simulink model "Induction_motor_drive"  (R2025a)
settings: Solver=ode45  StartTime=0.0  StopTime=1  RelTol=1e-3  EnableMultiTasking=on
libraries: spsIGBTDiodeLib x6, dspfdesign x3, spsCurrentMeasurementLib x3, spsVoltageMeasurementLib x3, spsGroundLib x1, simulink x1, spsDCVoltageSourceLib x1, sps_lib x1
settings Model: Creator=Cheku  LastModifiedBy=vijay
settings SolverCC: AlgebraicLoopSolver=TrustRegion
settings DataIOCC: LimitDataPoints=on  SaveFormat=Array  SignalLoggingSaveFormat=ModelDataLogs  ReturnWorkspaceOutputs=off
settings OptimizationCC: ExpressionDepthLimit=2147483647.0  InitFltsAndDblsToZero=on  LifeSpan=inf
settings DebuggingCC: UnderspecifiedInitializationDetection=Classic  MergeDetectMultiDrivingBlocksExec=none  SolverPrmCheckMsg=warning  FcnCallInpInsideContextMsg=warning  UnconnectedInputMsg=warning  UnconnectedOutputMsg=warning  UnconnectedLineMsg=warning  StateNameClashWarn=warning  SFUnexpectedBacktrackingDiag=warning  SFNoUnconditionalDefaultTransitionDiag=warning  SFExecutionAtInitializationDiag=none  ArithmeticOperatorsInVariantConditions=warning
settings HardwareCC: ProdBitPerPointer=32.0  ProdBitPerSizeT=32.0  ProdBitPerPtrDiffT=32.0  ProdLargestAtomicFloat=None  ProdIntDivRoundTo=Undefined  ProdEndianess=Unspecified  ProdWordSize=32.0  ProdHWDeviceType=32-bit Generic
settings ModelReferenceCC: PropagateSignalLabelsOutOfModel=off
settings SFSimCC: SimUseLocalCustomCode=off  CustomCodeUndefinedFunction=UseInterfaceOnly
settings RTWCC: RTWUseLocalCustomCode=off  GPUComputeCapability=3.5
settings CodeAppCC: StateflowObjectComments=on
settings GRTTargetCC: TargetLangStandard=C89/C90 (ANSI)  CombineOutputUpdateFcns=off  GRTInterface=on
settings ConfigComp: CovMetricSettings=dw  CovSaveCumulativeToWorkspaceVar=on  CovSaveSingleToWorkspaceVar=on  CovExternalEMLEnable=off

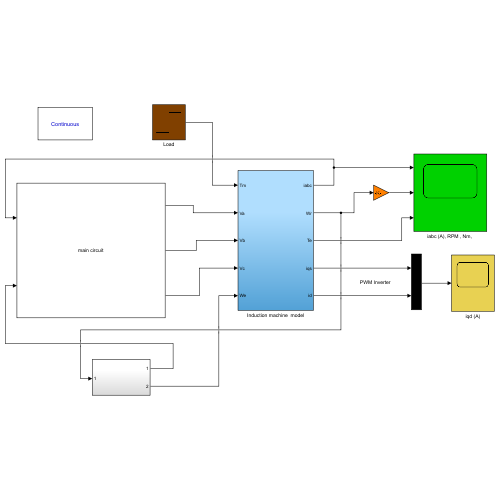
[thumbnail: Simulink's stored preview of the top-level diagram]
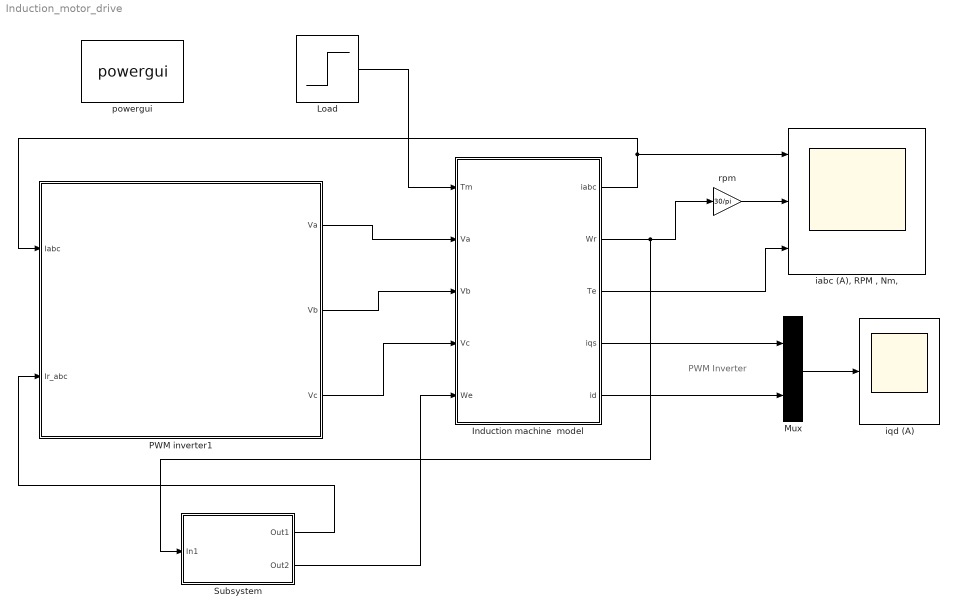
== system Induction_motor_drive ==
  note: PWM Inverter
  " rpm" : Gain  Gain=30/pi
  Induction machine  model : Subsystem
  Load : Step  Time=0  Before=0.025  After=5.00  SampleTime=0
  Mux : Mux  Inputs=2
  PWM inverter1 : Subsystem
      mask Display: disp('main circuit')
  Subsystem : Subsystem
  "iabc (A), RPM , Nm, " : Scope  NumInputPorts=3
      settings: TimeSpan=0.1  ActiveDisplayYMinimum=-681.97623  ActiveDisplayYMaximum=702.05177  DataLoggingVariableName=ScopeData9
  iqd (A) : Scope
      settings: ActiveDisplayYMinimum=-491.36775454277125  ActiveDisplayYMaximum=643.61004745722926  DataLoggingVariableName=ScopeData3
  powergui : sps_lib/powergui  SimulationMode=Continuous  SampleTime=50e-6  frequency=60  Iterations=50  frequencyindice=0  Pbase=100e6  ErrMax=1e-4  UnitsV=kV  UnitsW=MW  buscounter=0  FunctionMessages=off  echomessages=off  EnableUseOfTLC=off  CurrentSourceSwitches=on  DisableSnubberDevices=off  DisableRonSwitches=off  DisableVfSwitches=off  DisplayEquations=off  AutomaticDiscreteSolvers=off  SolverType=Tustin/Backward Euler (TBE)  Interpol=off  ExternalGateDelay=off  methode=off  Ts=0  x0status=blocks  SPID=off  SwTol=0  HookPort=off  NonlinearTolerance=1e-4  nMaxIteration=100  ContinueOnMaxIteration=off  RestoreLinks=warning  ResistiveCurrentMeasurement=off  Frange=[0:2:500]  Ylog=off  Xlog=on  ShowGrid=off  save=off  variable=ZData  structure=0  ZoomFFT=on  StartTime=0.0  cycles=1  DisplayStyle=1  fundamental=60  FreqAxis=off  MaxFrequency=1000  frequencyindicesteady=1  RmsSteady=1  display=off
  wires:
  PWM inverter1/1(Va) -> Induction machine  model/2(Va)
  Load/1 -> Induction machine  model/1(Tm)
  PWM inverter1/2(Vb) -> Induction machine  model/3(Vb)
  PWM inverter1/3(Vc) -> Induction machine  model/4(Vc)
  Subsystem/1(Out1) -> PWM inverter1/2(Ir_abc)
  Induction machine  model/1(iabc) -> "iabc (A), RPM , Nm, "/1, PWM inverter1/1(Iabc)
  Induction machine  model/2(Wr) -> Subsystem/1(In1), " rpm"/1
  Mux/1 -> iqd (A)/1
  Induction machine  model/4(iqs) -> Mux/1
  Induction machine  model/5(id) -> Mux/2
  Induction machine  model/3(Te) -> "iabc (A), RPM , Nm, "/3
  " rpm"/1 -> "iabc (A), RPM , Nm, "/2
  Subsystem/2(Out2) -> Induction machine  model/5(We)

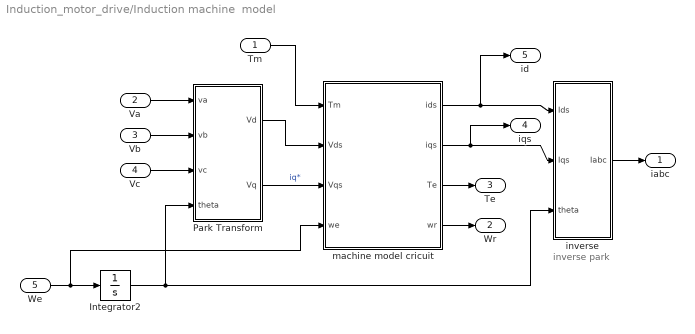
== system Induction_motor_drive/Induction machine  model ==
  note: inverse park
  Tm : Inport
  Va : Inport  Port=2
  Vb : Inport  Port=3
  Vc : Inport  Port=4
  We : Inport  Port=5
  Integrator2 : Integrator
  Park Transform : Subsystem
  "inverse " : Subsystem
  "machine model cricuit " : Subsystem
  iabc : Outport
  Wr : Outport  Port=2
  Te : Outport  Port=3
  iqs : Outport  Port=4
  id : Outport  Port=5
  wires:
  "machine model cricuit "/1(ids) -> "inverse "/1(Ids), id/1
  "machine model cricuit "/2(iqs) -> "inverse "/2(Iqs), iqs/1
  Park Transform/2(Vq) -> "machine model cricuit "/3(Vqs)  "iq*"
  Park Transform/1(Vd) -> "machine model cricuit "/2(Vds)
  Va/1 -> Park Transform/1(va)
  Vb/1 -> Park Transform/2(vb)
  Vc/1 -> Park Transform/3(vc)
  Tm/1 -> "machine model cricuit "/1(Tm)
  "inverse "/1(Iabc) -> iabc/1
  "machine model cricuit "/3(Te) -> Te/1
  We/1 -> Integrator2/1, "machine model cricuit "/4(we)
  "machine model cricuit "/4(wr) -> Wr/1
  Integrator2/1 -> "inverse "/3(theta), Park Transform/4(theta)

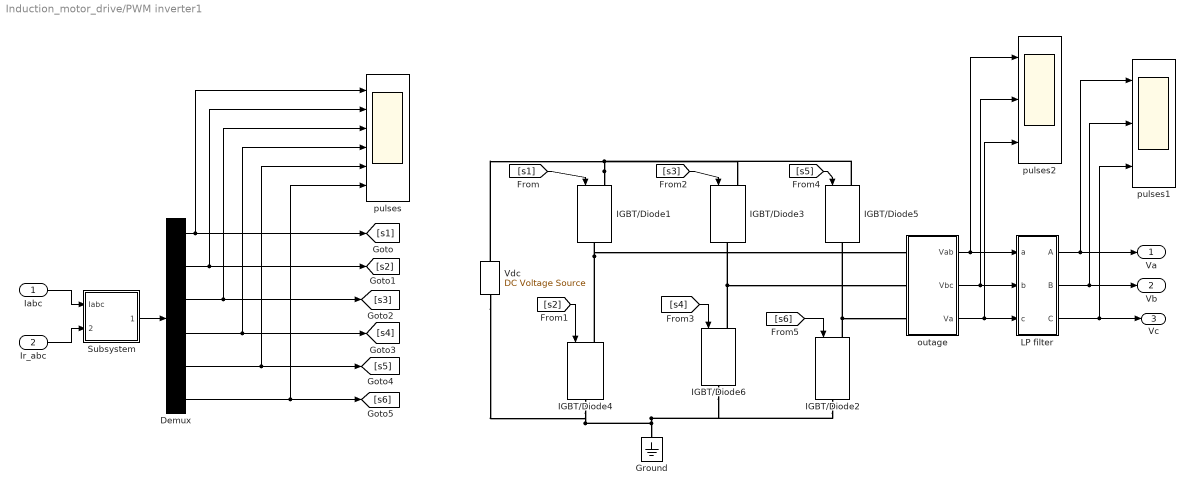
== system Induction_motor_drive/PWM inverter1 ==
  Iabc : Inport
  Ir_abc : Inport  Port=2
  Demux : Demux  Outputs=6
  Ground : spsGroundLib/Ground  LConnTagsString=a
  IGBT/Diode{1..6} (6 alike) : spsIGBTDiodeLib/IGBT//Diode  Ron=1e-3  Rs=1e5  Cs=inf  Measurements=off
  LP filter : Subsystem
  Subsystem : Subsystem
  Vdc : spsDCVoltageSourceLib/DC Voltage Source  Amplitude=283  Measurements=None
  outage : Subsystem
  pulses : Scope  NumInputPorts=6
      settings: ActiveDisplayYMinimum=-0.12499999999999997  ActiveDisplayYMaximum=1.125
  pulses1 : Scope  NumInputPorts=3
      settings: ActiveDisplayYMinimum=-143.13602  ActiveDisplayYMaximum=143.36169  DataLoggingVariableName=ScopeData2
  pulses2 : Scope  NumInputPorts=3
      settings: ActiveDisplayYMinimum=-353.74999292483255  ActiveDisplayYMaximum=353.74999292541224  DataLoggingVariableName=ScopeData4
  Va : Outport
  Vb : Outport  Port=2
  Vc : Outport  Port=3
  wires:
  Iabc/1 -> Subsystem/1(Iabc)
  Ir_abc/1 -> Subsystem/2(Ir_abc)
  Subsystem/1(pulses) -> Demux/1
  Demux/1 -> [s1], pulses/1
  [s1] -> IGBT/Diode1/1
  Demux/2 -> [s2], pulses/2
  [s2] -> IGBT/Diode4/1
  [s3] -> IGBT/Diode3/1
  Demux/3 -> [s3], pulses/3
  [s4] -> IGBT/Diode6/1
  Demux/4 -> [s4], pulses/4
  [s5] -> IGBT/Diode5/1
  [s6] -> IGBT/Diode2/1
  Demux/5 -> [s5], pulses/5
  Demux/6 -> [s6], pulses/6
  outage/1(Vab) -> LP filter/1(a), pulses2/1
  outage/2(Vbc) -> LP filter/2(b), pulses2/2
  outage/3(Va) -> LP filter/3(c), pulses2/3
  LP filter/1(A) -> Va/1, pulses1/1
  LP filter/2(B) -> Vb/1, pulses1/2
  LP filter/3(C) -> Vc/1, pulses1/3
  connections:
  IGBT/Diode1/LConn1 -- Vdc/RConn1 -- IGBT/Diode3/LConn1 -- IGBT/Diode5/LConn1
  IGBT/Diode4/LConn1 -- IGBT/Diode1/RConn1 -- outage/LConn1
  IGBT/Diode2/LConn1 -- IGBT/Diode5/RConn1 -- outage/LConn3
  Ground/LConn1 -- IGBT/Diode2/RConn1 -- IGBT/Diode6/RConn1 -- Vdc/LConn1 -- IGBT/Diode4/RConn1
  IGBT/Diode6/LConn1 -- outage/LConn2 -- IGBT/Diode3/RConn1

== system Induction_motor_drive/Subsystem ==
  In1 : Inport
  Integrator2 : Integrator
  Ref. Speed (rpm) : Constant  Value=1500
  "Ref. iabc " : Subsystem
  Sum : Sum  Inputs=+-  InputSameDT=on  SaturateOnIntegerOverflow=on  OutDataTypeStr=Inherit: Same as first input
  Sum2 : Sum
  Vector  control : Subsystem
  flux controller : Subsystem
  iqref1 : Subsystem  mask(PI Controller){I=2.5, P=5, sat=[ -30 30]}
      mask prompts: I "Integral"; P "Proportional:"; sat "Minimum and maximum outputs:"
      mask init:
      | min=sat(1);max=sat(2);
      mask Display: disp('PI')
  rad/sec : Gain  Gain=pi/30
  Out1 : Outport
  Out2 : Outport  Port=2
  wires:
  Ref. Speed (rpm)/1 -> rad/sec/1
  Sum/1 -> iqref1/1(In_1)
  rad/sec/1 -> Sum/1
  Vector  control/1(is*) -> "Ref. iabc "/1(is*)
  iqref1/1(Out_1) -> Vector  control/1(Te*)
  flux controller/1(Yr*) -> Vector  control/2(Yr)
  Sum2/1 -> Integrator2/1, Out2/1
  Integrator2/1 -> "Ref. iabc "/2(theta)
  Vector  control/2(wsl) -> Sum2/1
  In1/1 -> Sum2/2, Sum/2, flux controller/1(Wr)
  "Ref. iabc "/1(irabc) -> Out1/1

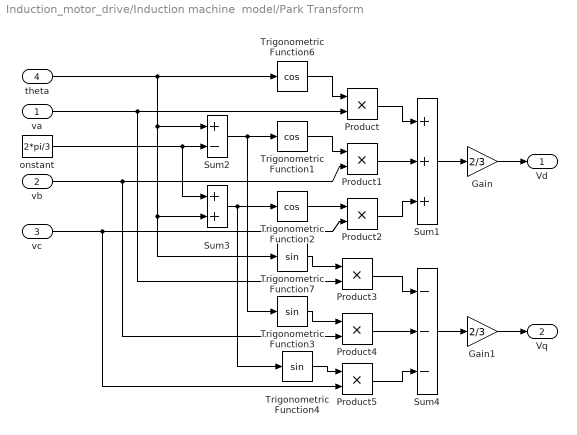
== system Induction_motor_drive/Induction machine  model/Park Transform ==
  va : Inport
  vb : Inport  Port=2
  vc : Inport  Port=3
  theta : Inport  Port=4
  Gain : Gain  Gain=2/3
  Gain1 : Gain  Gain=2/3
  Product{,1..5} (6 alike) : Product  RndMeth=Zero
  Sum1 : Sum  Inputs=+++  InputSameDT=on  SaturateOnIntegerOverflow=on  OutDataTypeStr=Inherit: Same as first input
  Sum2 : Sum  Inputs=+-  InputSameDT=on  SaturateOnIntegerOverflow=on  OutDataTypeStr=Inherit: Same as first input
  Sum3 : Sum  InputSameDT=on  SaturateOnIntegerOverflow=on  OutDataTypeStr=Inherit: Same as first input
  Sum4 : Sum  Inputs=---  InputSameDT=on  SaturateOnIntegerOverflow=on  OutDataTypeStr=Inherit: Same as first input
  Trigonometric Function1 : Trigonometry  Operator=cos
  Trigonometric Function2 : Trigonometry  Operator=cos
  Trigonometric Function3 : Trigonometry
  Trigonometric Function4 : Trigonometry
  Trigonometric Function6 : Trigonometry  Operator=cos
  Trigonometric Function7 : Trigonometry
  onstant : Constant  Value=2*pi/3
  Vd : Outport
  Vq : Outport  Port=2
  wires:
  Gain1/1 -> Vq/1
  Sum4/1 -> Gain1/1
  Product5/1 -> Sum4/3
  Trigonometric Function4/1 -> Product5/1
  Product4/1 -> Sum4/2
  Trigonometric Function3/1 -> Product4/1
  Product3/1 -> Sum4/1
  Trigonometric Function7/1 -> Product3/1
  Gain/1 -> Vd/1
  Sum1/1 -> Gain/1
  Product2/1 -> Sum1/3
  vc/1 -> Product5/2, Product2/2
  Trigonometric Function2/1 -> Product2/1
  Sum3/1 -> Trigonometric Function4/1, Trigonometric Function2/1
  Product1/1 -> Sum1/2
  vb/1 -> Product4/2, Product1/2
  Trigonometric Function1/1 -> Product1/1
  Sum2/1 -> Trigonometric Function3/1, Trigonometric Function1/1
  onstant/1 -> Sum3/1, Sum2/2
  Product/1 -> Sum1/1
  va/1 -> Product3/2, Product/2
  Trigonometric Function6/1 -> Product/1
  theta/1 -> Sum3/2, Trigonometric Function7/1, Sum2/1, Trigonometric Function6/1

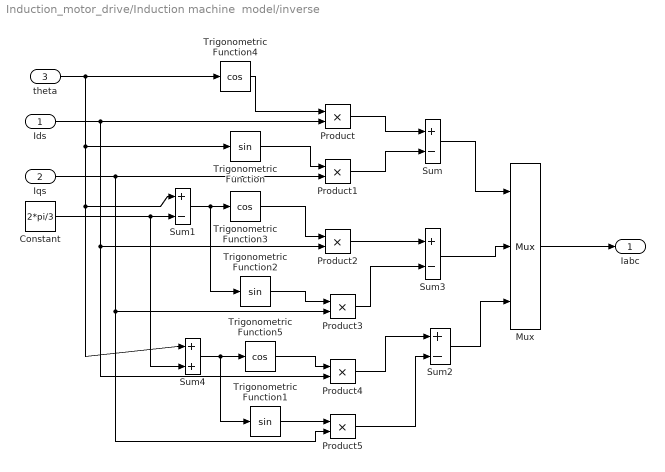
== system Induction_motor_drive/Induction machine  model/inverse  ==
  Ids : Inport
  Iqs : Inport  Port=2
  theta : Inport  Port=3
  Constant : Constant  Value=2*pi/3
  Mux : Mux  Inputs=3
  Product{,1..5} (6 alike) : Product  RndMeth=Zero
  Sum{,1..3} (4 alike) : Sum  Inputs=+-
  Sum4 : Sum  Inputs=|++
  Trigonometric Function : Trigonometry
  Trigonometric Function1 : Trigonometry
  Trigonometric Function2 : Trigonometry
  Trigonometric Function3 : Trigonometry  Operator=cos
  Trigonometric Function4 : Trigonometry  Operator=cos
  Trigonometric Function5 : Trigonometry  Operator=cos
  Iabc : Outport
  wires:
  Mux/1 -> Iabc/1
  Sum/1 -> Mux/1
  Sum3/1 -> Mux/2
  Sum2/1 -> Mux/3
  Product5/1 -> Sum2/2
  Product4/1 -> Sum2/1
  Trigonometric Function1/1 -> Product5/1
  Trigonometric Function5/1 -> Product4/1
  Sum4/1 -> Trigonometric Function1/1, Trigonometric Function5/1
  Product3/1 -> Sum3/2
  Trigonometric Function2/1 -> Product3/1
  Product2/1 -> Sum3/1
  Trigonometric Function3/1 -> Product2/1
  Sum1/1 -> Trigonometric Function2/1, Trigonometric Function3/1
  Constant/1 -> Sum4/2, Sum1/2
  Product1/1 -> Sum/2
  Product/1 -> Sum/1
  Iqs/1 -> Product5/2, Product3/2, Product1/2
  Trigonometric Function/1 -> Product1/1
  Ids/1 -> Product4/2, Product2/2, Product/2
  theta/1 -> Trigonometric Function/1, Sum4/1, Sum1/1, Trigonometric Function4/1
  Trigonometric Function4/1 -> Product/1

== system Induction_motor_drive/Induction machine  model/machine model cricuit  ==
  Tm : Inport
  Vds : Inport  Port=2
  Vqs : Inport  Port=3
  we : Inport  Port=4
  Saturation : Saturate  UpperLimit=5  LowerLimit=0
  Subsyste1 : Subsystem
  Subsystem : Subsystem
  Subsystem1 : Subsystem
  ids crt : Subsystem
  iqs crt : Subsystem
  ids : Outport
  iqs : Outport  Port=2
  Te : Outport  Port=3
  wr : Outport  Port=4
  wires:
  ids crt/1(ids) -> Subsystem/2(ids), Subsyste1/1(ids), iqs crt/4(ids), ids/1
  iqs crt/1(iqs) -> Subsystem/5(iqs), Subsystem1/4(iqs), ids crt/4(iqs), iqs/1
  Subsystem/2(wr) -> wr/1, iqs crt/6(Wr), ids crt/6(Wr), Subsyste1/3(Wr), Subsystem1/3(Wr)
  Subsystem1/1(Yqr) -> Subsystem/3(yqr), ids crt/2(Yqr), Subsyste1/4(Yqr), iqs crt/3(Yqr)
  Subsyste1/1(Ydr) -> ids crt/3(Ydr), Subsystem1/1(Ydr), Subsystem/4(ydr), iqs crt/2(Ydr)
  Tm/1 -> Subsystem/1(TM)
  we/1 -> Subsyste1/2(We), ids crt/5(We), Subsystem1/2(We), iqs crt/5(We)
  Vqs/1 -> iqs crt/1(Vqs)
  Vds/1 -> ids crt/1(Vds)
  Subsystem/1(Te) -> Saturation/1
  Saturation/1 -> Te/1

== system Induction_motor_drive/PWM inverter1/LP filter ==
  a : Inport
  b : Inport  Port=2
  c : Inport  Port=3
  Analog Filter Desg : dspfdesign/Analog Filter Design  method=Butterworth  filttype=Lowpass  N=3  Wlo=12566.3706  Whi=80  Rp=3  Rs=5
  Analog Filter Desg1 : dspfdesign/Analog Filter Design  method=Butterworth  filttype=Lowpass  N=3  Wlo=12566.3706  Whi=80  Rp=3  Rs=5
  Analog Filter Desg2 : dspfdesign/Analog Filter Design  method=Butterworth  filttype=Lowpass  N=3  Wlo=12566.3706  Whi=80  Rp=3  Rs=5
  A : Outport
  B : Outport  Port=2
  C : Outport  Port=3
  wires:
  a/1 -> Analog Filter Desg/1
  Analog Filter Desg/1 -> A/1
  b/1 -> Analog Filter Desg1/1
  Analog Filter Desg1/1 -> B/1
  c/1 -> Analog Filter Desg2/1
  Analog Filter Desg2/1 -> C/1

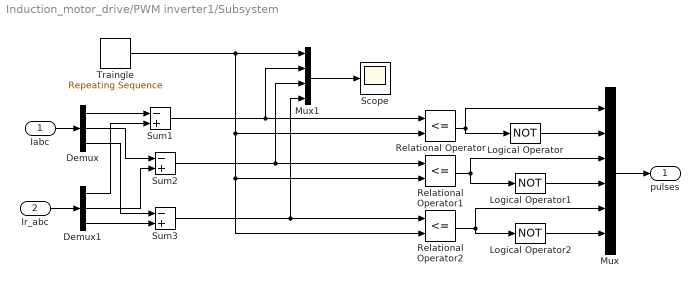
== system Induction_motor_drive/PWM inverter1/Subsystem ==
  Iabc : Inport
  Ir_abc : Inport  Port=2
  Demux : Demux  Outputs=3
  Demux1 : Demux  Outputs=3
  Logical Operator : Logic  Operator=NOT
  Logical Operator1 : Logic  Operator=NOT
  Logical Operator2 : Logic  Operator=NOT
  Mux : Mux  Inputs=6
  Mux1 : Mux
  Relational Operator : RelationalOperator  Operator=<=  OutDataTypeStr=boolean  InputSameDT=off
  Relational Operator1 : RelationalOperator  Operator=<=  OutDataTypeStr=boolean  InputSameDT=off
  Relational Operator2 : RelationalOperator  Operator=<=  OutDataTypeStr=boolean  InputSameDT=off
  Scope : Scope
      settings: ActiveDisplayYMinimum=-124.55267  ActiveDisplayYMaximum=124.74286  DataLoggingVariableName=ScopeData11
  Sum1 : Sum  Inputs=-+  InputSameDT=on  SaturateOnIntegerOverflow=on  OutDataTypeStr=Inherit: Same as first input
  Sum2 : Sum  Inputs=-+  InputSameDT=on  SaturateOnIntegerOverflow=on  OutDataTypeStr=Inherit: Same as first input
  Sum3 : Sum  Inputs=-+  InputSameDT=on  SaturateOnIntegerOverflow=on  OutDataTypeStr=Inherit: Same as first input
  Traingle : simulink/Sources/Repeating Sequence  rep_seq_t=[0 1/2000/4 3/2000/4 1/2000]  rep_seq_y="[0 -100  100  0]"
  pulses : Outport
  wires:
  Iabc/1 -> Demux/1
  Ir_abc/1 -> Demux1/1
  Demux/1 -> Sum1/1
  Demux1/1 -> Sum1/2
  Demux/2 -> Sum2/1
  Demux1/2 -> Sum2/2
  Demux/3 -> Sum3/1
  Demux1/3 -> Sum3/2
  Relational Operator/1 -> Logical Operator/1, Mux/1
  Logical Operator/1 -> Mux/2
  Relational Operator1/1 -> Mux/3, Logical Operator1/1
  Logical Operator1/1 -> Mux/4
  Relational Operator2/1 -> Logical Operator2/1, Mux/5
  Logical Operator2/1 -> Mux/6
  Mux/1 -> pulses/1
  Sum1/1 -> Relational Operator/1, Mux1/2
  Sum2/1 -> Relational Operator1/1, Mux1/3
  Sum3/1 -> Relational Operator2/1, Mux1/4
  Traingle/1 -> Relational Operator2/2, Relational Operator1/2, Relational Operator/2, Mux1/1
  Mux1/1 -> Scope/1

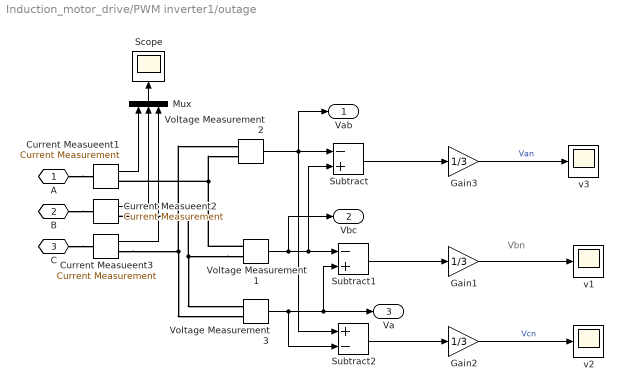
== system Induction_motor_drive/PWM inverter1/outage ==
  note: Vbn
  Current Measueent1 : spsCurrentMeasurementLib/Current Measurement  PhasorSimulation=off  OutputType=Complex  PSBequivalent=0
  Current Measueent2 : spsCurrentMeasurementLib/Current Measurement  PhasorSimulation=off  OutputType=Complex  PSBequivalent=0
  Current Measueent3 : spsCurrentMeasurementLib/Current Measurement  PhasorSimulation=off  OutputType=Complex  PSBequivalent=0
  Gain1 : Gain  Gain=1/3
  Gain2 : Gain  Gain=1/3
  Gain3 : Gain  Gain=1/3
  Mux : Mux  Inputs=3
  Scope : Scope
      settings: ActiveDisplayYMinimum=-3.1169527740766263  ActiveDisplayYMaximum=1.936947616674654
  Subtract : Sum  Inputs=-+
  Subtract1 : Sum  Inputs=-+
  Subtract2 : Sum  Inputs=+-
  Voltage Measurement1 : spsVoltageMeasurementLib/Voltage Measurement  PhasorSimulation=off  OutputType=Complex  PSBequivalent=0
  Voltage Measurement2 : spsVoltageMeasurementLib/Voltage Measurement  PhasorSimulation=off  OutputType=Complex  PSBequivalent=0
  Voltage Measurement3 : spsVoltageMeasurementLib/Voltage Measurement  PhasorSimulation=off  OutputType=Complex  PSBequivalent=0
  v1 : Scope
      settings: ActiveDisplayYMinimum=-283.8728707821619  ActiveDisplayYMaximum=262.14024076146268  DataLoggingVariableName=ScopeData25
  v2 : Scope
      settings: ActiveDisplayYMinimum=-235.8333276306908  ActiveDisplayYMaximum=235.83332850733069  DataLoggingVariableName=ScopeData26
  v3 : Scope
      settings: ActiveDisplayYMinimum=-286.94561491531204  ActiveDisplayYMaximum=259.06749789646426  DataLoggingVariableName=ScopeData27
  A : PMIOPort  Side=Left
  B : PMIOPort  Port=2  Side=Left
  C : PMIOPort  Port=3  Side=Left
  Vab : Outport
  Vbc : Outport  Port=2
  Va : Outport  Port=3
  wires:
  Voltage Measurement2/1 -> Subtract/1, Subtract2/1, Vab/1
  Voltage Measurement1/1 -> Subtract/2, Subtract1/1, Vbc/1
  Current Measueent1/1 -> Mux/1
  Current Measueent2/1 -> Mux/2
  Current Measueent3/1 -> Mux/3
  Mux/1 -> Scope/1
  Subtract/1 -> Gain3/1
  Gain3/1 -> v3/1  "Van"
  Voltage Measurement3/1 -> Subtract2/2, Subtract1/2, Va/1
  Subtract1/1 -> Gain1/1
  Gain1/1 -> v1/1
  Subtract2/1 -> Gain2/1
  Gain2/1 -> v2/1  "Vcn"
  connections:
  Voltage Measurement1/LConn1 -- Current Measueent1/RConn1 -- Voltage Measurement2/LConn2
  Voltage Measurement1/LConn2 -- Current Measueent2/RConn1 -- Voltage Measurement3/LConn1
  Current Measueent3/RConn1 -- Voltage Measurement2/LConn1 -- Voltage Measurement3/LConn2
  A/RConn1 -- Current Measueent1/LConn1
  B/RConn1 -- Current Measueent2/LConn1
  C/RConn1 -- Current Measueent3/LConn1

== system Induction_motor_drive/Subsystem/Ref. iabc  ==
  is* : Inport
  theta : Inport  Port=2
  Constant : Constant  Value=2*pi/3
  Mux1 : Mux  Inputs=3
  Product2 : Product  InputSameDT=on  RndMeth=Zero  SaturateOnIntegerOverflow=on  OutDataTypeStr=Inherit: Same as first input
  Product4 : Product  InputSameDT=on  RndMeth=Zero  SaturateOnIntegerOverflow=on  OutDataTypeStr=Inherit: Same as first input
  Product7 : Product  InputSameDT=on  RndMeth=Zero  SaturateOnIntegerOverflow=on  OutDataTypeStr=Inherit: Same as first input
  Sum2 : Sum  Inputs=+-  InputSameDT=on  SaturateOnIntegerOverflow=on  OutDataTypeStr=Inherit: Same as first input
  Sum4 : Sum  InputSameDT=on  SaturateOnIntegerOverflow=on  OutDataTypeStr=Inherit: Same as first input
  Trigonometric Function1 : Trigonometry  Operator=cos
  Trigonometric Function3 : Trigonometry  Operator=cos
  Trigonometric Function6 : Trigonometry  Operator=cos
  irabc : Outport
  wires:
  theta/1 -> Trigonometric Function6/1, Sum2/1, Sum4/1
  Trigonometric Function6/1 -> Product7/1
  is*/1 -> Product7/2, Product2/2, Product4/2
  Product7/1 -> Mux1/1
  Sum2/1 -> Trigonometric Function1/1
  Trigonometric Function1/1 -> Product2/1
  Product2/1 -> Mux1/2
  Sum4/1 -> Trigonometric Function3/1
  Trigonometric Function3/1 -> Product4/1
  Product4/1 -> Mux1/3
  Mux1/1 -> irabc/1
  Constant/1 -> Sum2/2, Sum4/2

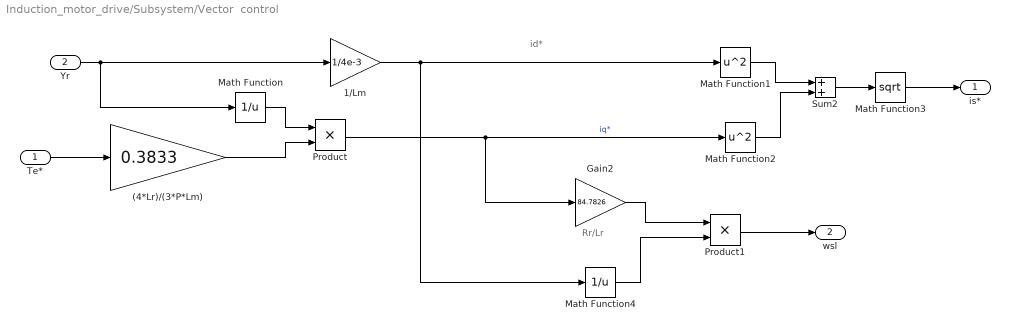
== system Induction_motor_drive/Subsystem/Vector  control ==
  note: id*
  note: Rr/Lr
  Te* : Inport
  Yr : Inport  Port=2
  (4*Lr)/(3*P*Lm) : Gain  Gain=0.3833
  1/Lm : Gain  Gain=1/4e-3
  Gain2 : Gain  Gain=84.7826
  Math Function : Math  Operator=reciprocal  SignedPower=on
  Math Function1 : Math  Operator=square  SignedPower=on
  Math Function2 : Math  Operator=square  SignedPower=on
  Math Function3 : Math  Operator=sqrt  SignedPower=on
  Math Function4 : Math  Operator=reciprocal  SignedPower=on
  Product : Product  RndMeth=Zero
  Product1 : Product  RndMeth=Zero
  Sum2 : Sum
  is* : Outport
  wsl : Outport  Port=2
  wires:
  Yr/1 -> 1/Lm/1, Math Function/1
  Te*/1 -> (4*Lr)/(3*P*Lm)/1
  (4*Lr)/(3*P*Lm)/1 -> Product/2
  Math Function/1 -> Product/1
  Math Function1/1 -> Sum2/1
  Math Function2/1 -> Sum2/2
  Sum2/1 -> Math Function3/1
  Math Function3/1 -> is*/1
  Product/1 -> Gain2/1, Math Function2/1  "iq*"
  1/Lm/1 -> Math Function1/1, Math Function4/1
  Gain2/1 -> Product1/1
  Math Function4/1 -> Product1/2
  Product1/1 -> wsl/1

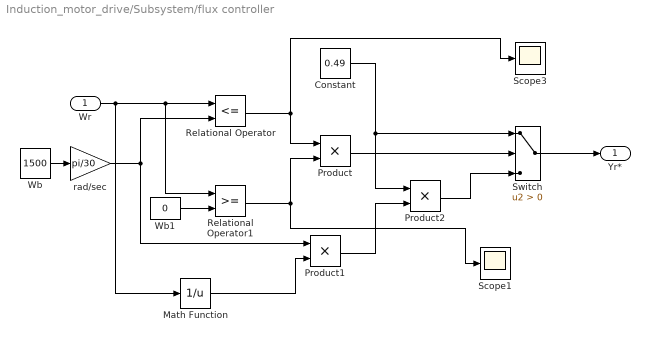
== system Induction_motor_drive/Subsystem/flux controller ==
  Wr : Inport
  Constant : Constant  Value=0.49
  Math Function : Math  Operator=reciprocal  SignedPower=on
  Product : Product  RndMeth=Zero
  Product1 : Product  RndMeth=Zero
  Product2 : Product  RndMeth=Zero
  Relational Operator : RelationalOperator  Operator=<=  OutDataTypeStr=boolean  InputSameDT=off
  Relational Operator1 : RelationalOperator  OutDataTypeStr=boolean  InputSameDT=off
  Scope1 : Scope
      settings: ActiveDisplayYMinimum=-55  ActiveDisplayYMaximum=55  DataLoggingVariableName=ScopeData8
  Scope3 : Scope
      settings: ActiveDisplayYMinimum=-55  ActiveDisplayYMaximum=55  DataLoggingVariableName=ScopeData7
  Switch : Switch  Criteria=u2 > Threshold  SaturateOnIntegerOverflow=off  InputSameDT=off
  Wb : Constant  Value=1500
  Wb1 : Constant  Value=0
  rad/sec : Gain  Gain=pi/30
  Yr* : Outport
  wires:
  Relational Operator/1 -> Product/1, Scope3/1
  Relational Operator1/1 -> Product/2, Scope1/1
  Wr/1 -> Relational Operator/1, Relational Operator1/1, Math Function/1
  Wb/1 -> rad/sec/1
  Product/1 -> Switch/2
  Constant/1 -> Switch/1, Product2/1
  Math Function/1 -> Product1/2
  Product1/1 -> Product2/2
  Product2/1 -> Switch/3
  Switch/1 -> Yr*/1
  Wb1/1 -> Relational Operator1/2
  rad/sec/1 -> Relational Operator/2, Product1/1

== system Induction_motor_drive/Subsystem/iqref1 ==
  In_1 : Inport
  Integral : TransferFcn  Numerator=[I]  Denominator=[1 0]
  Proportional : Gain  Gain=P  SaturateOnIntegerOverflow=on  OutDataTypeStr=Inherit: Same as input  ParamDataTypeStr=Inherit: Same as input
  Saturation : Saturate  UpperLimit=max  LowerLimit=min
  Sum : Sum  InputSameDT=on  SaturateOnIntegerOverflow=on  OutDataTypeStr=Inherit: Same as first input
  Out_1 : Outport  InitialOutput=0
  wires:
  Integral/1 -> Sum/2
  In_1/1 -> Integral/1, Proportional/1
  Proportional/1 -> Sum/1
  Sum/1 -> Saturation/1
  Saturation/1 -> Out_1/1

== system Induction_motor_drive/Induction machine  model/machine model cricuit /Subsyste1 ==
  note: C6 = Lm*Rr/Lr
  note: C5 = Rr/Lr
  ids : Inport
  We : Inport  Port=2
  Wr : Inport  Port=3
  Yqr : Inport  Port=4
  Add1 : Sum  Inputs=++-
  Gain4 : Gain  Gain=0.3391
  Integrator : Integrator
  Product : Product  RndMeth=Zero
  Subtract : Sum  Inputs=+-
  ain3 : Gain  Gain=84.7826
  Ydr : Outport
  wires:
  Product/1 -> Add1/2
  Yqr/1 -> Product/2
  Wr/1 -> Subtract/2
  We/1 -> Subtract/1
  Subtract/1 -> Product/1
  Gain4/1 -> Add1/1
  Add1/1 -> Integrator/1
  Integrator/1 -> Ydr/1, ain3/1
  ain3/1 -> Add1/3
  ids/1 -> Gain4/1

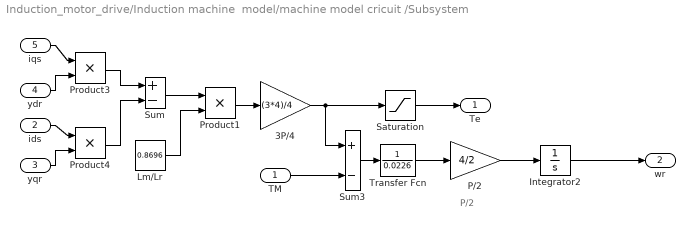
== system Induction_motor_drive/Induction machine  model/machine model cricuit /Subsystem ==
  note: P/2
  TM : Inport
  ids : Inport  Port=2
  yqr : Inport  Port=3
  ydr : Inport  Port=4
  iqs : Inport  Port=5
  3P/4 : Gain  Gain=(3*4)/4
  Integrator2 : Integrator
  Lm/Lr : Constant  Value=0.8696
  P/2 : Gain  Gain=4/2
  Product1 : Product  RndMeth=Zero
  Product3 : Product  RndMeth=Zero
  Product4 : Product  RndMeth=Zero
  Saturation : Saturate  UpperLimit=20  LowerLimit=-20
  Sum : Sum  Inputs=+-
  Sum3 : Sum  Inputs=+-
  Transfer Fcn : TransferFcn  Denominator=[0.0226]
  Te : Outport
  wr : Outport  Port=2
  wires:
  Transfer Fcn/1 -> P/2/1
  Integrator2/1 -> wr/1
  yqr/1 -> Product4/2
  ids/1 -> Product4/1
  ydr/1 -> Product3/2
  iqs/1 -> Product3/1
  TM/1 -> Sum3/2
  P/2/1 -> Integrator2/1
  Sum3/1 -> Transfer Fcn/1
  Product4/1 -> Sum/2
  Product3/1 -> Sum/1
  3P/4/1 -> Sum3/1, Saturation/1
  Product1/1 -> 3P/4/1
  Sum/1 -> Product1/1
  Lm/Lr/1 -> Product1/2
  Saturation/1 -> Te/1

== system Induction_motor_drive/Induction machine  model/machine model cricuit /Subsystem1 ==
  note: C6 = Lm*Rr/Lr
  note: C6 = Lm*Rr/Lr
  Ydr : Inport
  We : Inport  Port=2
  Wr : Inport  Port=3
  iqs : Inport  Port=4
  Add1 : Sum  Inputs=+--
  Gain4 : Gain  Gain=0.3391
  Integrator : Integrator
  Product : Product  RndMeth=Zero
  Subtract : Sum  Inputs=+-
  ain3 : Gain  Gain=84.7826
  Yqr : Outport
  wires:
  Product/1 -> Add1/2
  Ydr/1 -> Product/2
  Subtract/1 -> Product/1
  Gain4/1 -> Add1/1
  Add1/1 -> Integrator/1
  Integrator/1 -> Yqr/1, ain3/1
  ain3/1 -> Add1/3
  iqs/1 -> Gain4/1
  Wr/1 -> Subtract/2
  We/1 -> Subtract/1

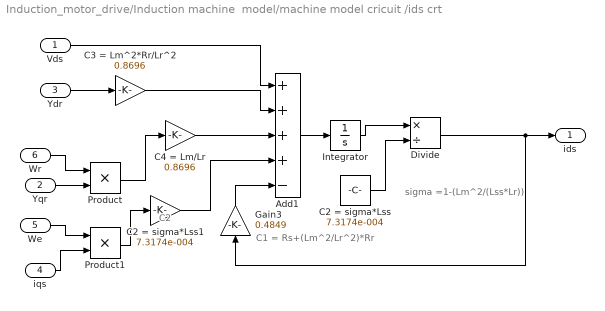
== system Induction_motor_drive/Induction machine  model/machine model cricuit /ids crt ==
  note: C1 = Rs+(Lm^2/Lr^2)*Rr
  note: sigma =1-(Lm^2/(Lss*Lr))
  note: C2
  Vds : Inport
  Yqr : Inport  Port=2
  Ydr : Inport  Port=3
  iqs : Inport  Port=4
  We : Inport  Port=5
  Wr : Inport  Port=6
  Add1 : Sum  Inputs=++++-
  C2 = sigma*Lss : Constant  Value=7.3174e-004
  C2 = sigma*Lss1 : Gain  Gain=7.3174e-004
  C3 = Lm^2*Rr/Lr^2 : Gain  Gain=0.8696
  C4 = Lm/Lr : Gain  Gain=0.8696
  Divide : Product  Inputs=*/
  Gain3 : Gain  Gain=0.4849
  Integrator : Integrator
  Product : Product  RndMeth=Zero
  Product1 : Product  RndMeth=Zero
  ids : Outport
  wires:
  Vds/1 -> Add1/1
  Ydr/1 -> C3 = Lm^2*Rr/Lr^2/1
  C3 = Lm^2*Rr/Lr^2/1 -> Add1/2
  Product/1 -> C4 = Lm/Lr/1
  Yqr/1 -> Product/2
  Wr/1 -> Product/1
  C4 = Lm/Lr/1 -> Add1/3
  iqs/1 -> Product1/2
  We/1 -> Product1/1
  Product1/1 -> C2 = sigma*Lss1/1
  C2 = sigma*Lss1/1 -> Add1/4
  Gain3/1 -> Add1/5
  Divide/1 -> Gain3/1, ids/1
  Integrator/1 -> Divide/1
  Add1/1 -> Integrator/1
  C2 = sigma*Lss/1 -> Divide/2

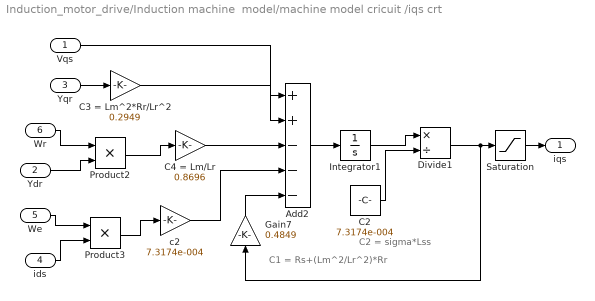
== system Induction_motor_drive/Induction machine  model/machine model cricuit /iqs crt ==
  note: C2 = sigma*Lss
  note: C1 = Rs+(Lm^2/Lr^2)*Rr
  Vqs : Inport
  Ydr : Inport  Port=2
  Yqr : Inport  Port=3
  ids : Inport  Port=4
  We : Inport  Port=5
  Wr : Inport  Port=6
  Add2 : Sum  Inputs=++---
  C2 : Constant  Value=7.3174e-004
  C3 = Lm^2*Rr/Lr^2 : Gain  Gain=0.2949
  C4 = Lm/Lr : Gain  Gain=0.8696
  Divide1 : Product  Inputs=*/
  Gain7 : Gain  Gain=0.4849
  Integrator1 : Integrator
  Product2 : Product  RndMeth=Zero
  Product3 : Product  RndMeth=Zero
  Saturation : Saturate  UpperLimit=300  LowerLimit=-300
  c2 : Gain  Gain=7.3174e-004
  iqs : Outport
  wires:
  Vqs/1 -> Add2/1
  Yqr/1 -> C3 = Lm^2*Rr/Lr^2/1
  C3 = Lm^2*Rr/Lr^2/1 -> Add2/2
  Product2/1 -> C4 = Lm/Lr/1
  Ydr/1 -> Product2/2
  Wr/1 -> Product2/1
  C4 = Lm/Lr/1 -> Add2/3
  ids/1 -> Product3/2
  We/1 -> Product3/1
  Product3/1 -> c2/1
  c2/1 -> Add2/4
  Gain7/1 -> Add2/5
  Divide1/1 -> Gain7/1, Saturation/1
  Integrator1/1 -> Divide1/1
  Add2/1 -> Integrator1/1
  C2/1 -> Divide1/2
  Saturation/1 -> iqs/1
